simulink model "functions_for_different_time_intervals"  (R2021a)
settings: Solver=FixedStepAuto  StartTime=-9  StopTime=9  FixedStep=0.5  RelTol=1e-3
settings Model: Creator=Acer  LastModifiedBy=Acer

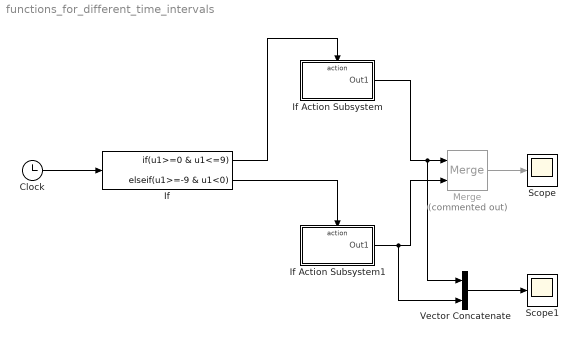
== system functions_for_different_time_intervals ==
  Clock : Clock
  If : If  IfExpression=u1>=0 & u1<=9  ElseIfExpressions=u1>=-9 & u1<0  ShowElse=off
  If Action Subsystem : Subsystem  TreatAsAtomicUnit=on
  If Action Subsystem1 : Subsystem  TreatAsAtomicUnit=on
  Merge : Merge  Commented=on
  Scope : Scope
  Scope1 : Scope
  Vector Concatenate : Concatenate
  wires:
  Clock/1 -> If/1
  If/1 -> If Action Subsystem/Action
  If/2 -> If Action Subsystem1/Action
  If Action Subsystem1/1(Out1) -> Vector Concatenate/2, Merge/2
  If Action Subsystem/1(Out1) -> Vector Concatenate/1, Merge/1
  Merge/1 -> Scope/1
  Vector Concatenate/1 -> Scope1/1

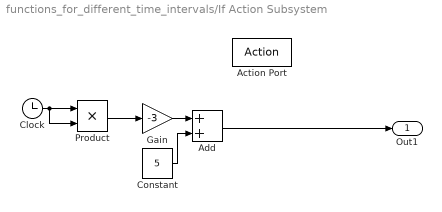
== system functions_for_different_time_intervals/If Action Subsystem ==
  Action Port : ActionPort  ActionPortLabel=if(u1>=0 & u1<=9)
  Add : Sum
  Clock : Clock
  Constant : Constant  Value=5
  Gain : Gain  Gain=-3
  Product : Product
  Out1 : Outport
  wires:
  Clock/1 -> Product/2, Product/1
  Product/1 -> Gain/1
  Gain/1 -> Add/1
  Constant/1 -> Add/2
  Add/1 -> Out1/1

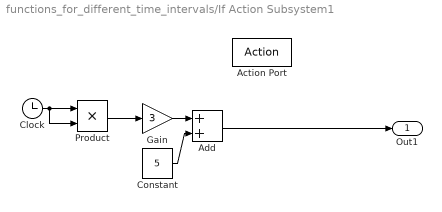
== system functions_for_different_time_intervals/If Action Subsystem1 ==
  Action Port : ActionPort  ActionPortLabel=elseif(u1>=-9 & u1<0)
  Add : Sum
  Clock : Clock
  Constant : Constant  Value=5
  Gain : Gain  Gain=3
  Product : Product
  Out1 : Outport
  wires:
  Add/1 -> Out1/1
  Constant/1 -> Add/2
  Gain/1 -> Add/1
  Product/1 -> Gain/1
  Clock/1 -> Product/1, Product/2
